simulink model "modulacaoqpsk-2"  (R2015a)
settings: Solver=FixedStepDiscrete  StartTime=0.0  StopTime=10.0  RelTol=1e-3
libraries: dspsigops x2, simulink x1, commdigbbndpm3 x1
settings Model: Creator=jessica.c13  LastModifiedBy=aluno
settings OptimizationCC: BlockReduction=off  ConditionallyExecuteInputs=off  InlineParams=on
settings DebuggingCC: AlgebraicLoopMsg=error
settings HardwareCC: ProdHWDeviceType=ASIC/FPGA->ASIC/FPGA  ProdEqTarget=off

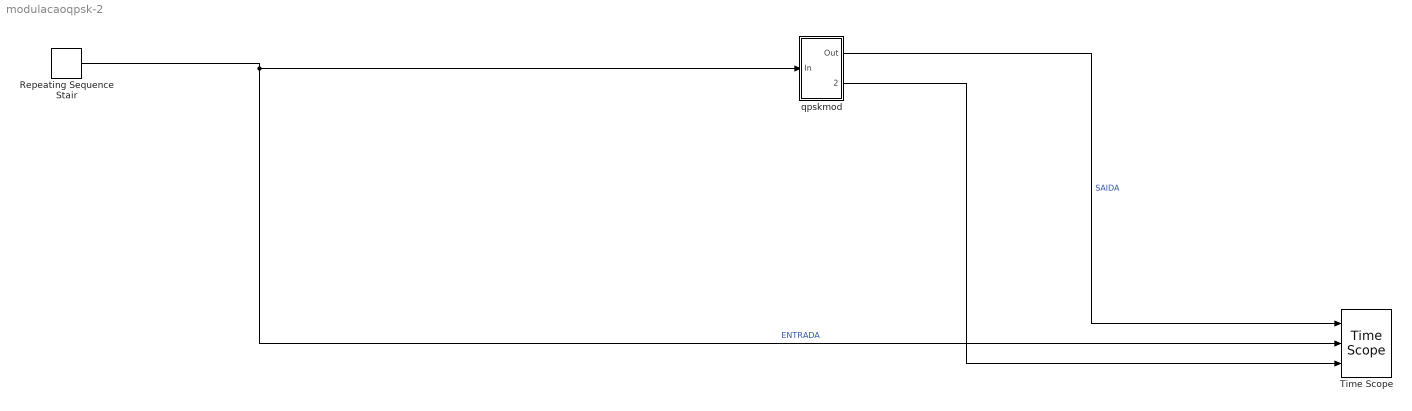
== system modulacaoqpsk-2 ==
  Repeating Sequence Stair : simulink/Sources/Repeating Sequence Stair  OutValues=[0 0 0 0 0 0 0 0 0 0 0 0 0 0 0 0 0 0 0 0 0 0 0 0 0 0 0 0 0 0 0 0 0 0 0 0 0 0 0 0 0 0 0 0 0 0 0 0 0 0 1 1 1 1 1 1 1 1 1 1 1 1 1 1 1 1 1 1 1 1 1 1 1 1 1 1 1 1 1 1 1 1 1 1 1 1 1 1 1 1 1 1 1 1 1 1 1 1 1 1 2 2 2 2 2 2 2 2 2 2 2 2 2 2 2 2 2 2 2 2 2 2 2 2 2 2 2 2 2 2 2 2 2 2 2 2 2 2 2 2 2 2 2 2 2 2 2 2 2 2 3 3 3 3 3 3 3 3 3 3 3 3 3 3 3 3 3 3 3 3 3 3 3 3 3 3 3 3 3 3 3 3 3 3 3 3 3 3 3 3 3 3 3 3 3 3 3 3 3 3].'  tsamp=1/100  OutMin=0  OutMax=3  OutDataTypeStr=int8  OutputDataTypeScalingMode=int8  OutDataType=fixdt(0,8)  ConRadixGroup=Best Precision: Vector-wise  OutScaling=2^-12
  Time Scope : TimeScope  DefaultConfigurationName=spbscopes.TimeScopeBlockCfg  NumInputPorts=3
  qpskmod : Subsystem
  wires:
  Repeating Sequence Stair/1 -> qpskmod/1(In), Time Scope/2  "ENTRADA"
  qpskmod/1(Out) -> Time Scope/1  "SAIDA"
  qpskmod/2(Out1) -> Time Scope/3

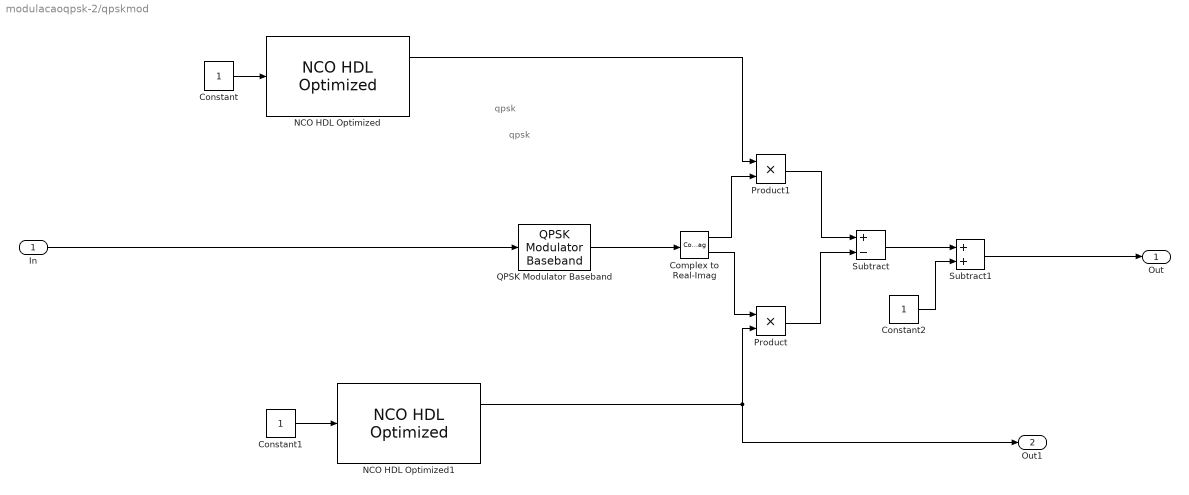
== system modulacaoqpsk-2/qpskmod ==
  note: qpsk
  note: qpsk
  In : Inport
  Complex to Real-Imag : ComplexToRealImag
  Constant : Constant  OutDataTypeStr=boolean
  Constant1 : Constant  OutDataTypeStr=boolean
  Constant2 : Constant  OutDataTypeStr=Inherit: Inherit via back propagation  SampleTime=1/100
  NCO HDL Optimized : dspsigops/NCO HDL Optimized  PhaseIncrementSource=Property  PhaseIncrement=4096  PhaseOffsetSource=Property  PhaseOffset=0  DitherSource=Property  NumDitherBits=4  PhaseQuantization=on  NumQuantizerAccumulatorBits=12  LUTCompress=off  ResetAction=off  Waveform=Cosine  PhasePort=off  AccumulatorWL=16  OutputDataType=Binary point scaling  OutputWL=16  OutputFL=14  SimulateUsing=Code generation
  NCO HDL Optimized1 : dspsigops/NCO HDL Optimized  PhaseIncrementSource=Property  PhaseIncrement=4096  PhaseOffsetSource=Property  PhaseOffset=0  DitherSource=Property  NumDitherBits=4  PhaseQuantization=on  NumQuantizerAccumulatorBits=12  LUTCompress=off  ResetAction=off  Waveform=Sine  PhasePort=off  AccumulatorWL=16  OutputDataType=Binary point scaling  OutputWL=16  OutputFL=14  SimulateUsing=Interpreted execution
  Product : Product
  Product1 : Product
  QPSK Modulator Baseband : commdigbbndpm3/QPSK Modulator Baseband  InType=Integer  Enc=Gray  Ph=0  outDtype=Fixed-point  outWordLen=8  outUDDataType=sfix(16)  outFracLenMode=Best precision  outFracLen=15
  Subtract : Sum  Inputs=+-  OutDataTypeStr=Inherit: Inherit via back propagation
  Subtract1 : Sum  OutDataTypeStr=fixdt(0,12,10)
  Out : Outport
  Out1 : Outport  Port=2
  wires:
  Constant1/1 -> NCO HDL Optimized1/1
  Constant/1 -> NCO HDL Optimized/1
  In/1 -> QPSK Modulator Baseband/1
  Product1/1 -> Subtract/1
  NCO HDL Optimized1/1 -> Product/2, Out1/1
  NCO HDL Optimized/1 -> Product1/1
  Complex to Real-Imag/2 -> Product/1
  QPSK Modulator Baseband/1 -> Complex to Real-Imag/1
  Complex to Real-Imag/1 -> Product1/2
  Product/1 -> Subtract/2
  Subtract1/1 -> Out/1
  Subtract/1 -> Subtract1/1
  Constant2/1 -> Subtract1/2
